simulink model "ControlVehiculoV"  (R2023b)
settings: Solver=FixedStepAuto  StartTime=0.0  StopTime=10  RelTol=1e-3  EnableMultiTasking=on
model workspace (MAT data in the model file):
  d = 0.223
settings Model: ExtModeTrigDuration=2  Creator=Manuel  LastModifiedBy=Manuel
settings OptimizationCC: EnhancedBackFolding=on  PassReuseOutputArgsAs=Individual arguments  ZeroExternalMemoryAtStartup=off  ZeroInternalMemoryAtStartup=off  MaxStackSize=64  OptimizeBlockOrder=speed  DifferentSizesBufferReuse=on  OptimizationCustomize=off  EfficientTunableParamExpr=on
settings DebuggingCC: ParameterTunabilityLossMsg=error
settings HardwareCC: ProdBitPerInt=16  ProdBitPerPointer=16  ProdBitPerSizeT=16  ProdBitPerPtrDiffT=16  ProdLargestAtomicFloat=None  ProdWordSize=8  ProdHWDeviceType=Atmel->AVR
settings SFSimCC: MATLABDynamicMemAlloc=off
settings RTWCC: Description=Embedded Coder  SystemTargetFile=ert.tlc  HardwareBoard=Arduino Mega 2560  TemplateMakefile=ert_default_tmf  Toolchain=Arduino AVR  BuildConfiguration=Faster Runs
settings CodeAppCC: ForceParamTrailComments=on  IgnoreCustomStorageClasses=off  OperatorAnnotations=on  SimulinkDataObjDesc=on  SFDataObjDesc=on  InsertBlockDesc=on
settings ERTTargetCC: SupportContinuousTime=on  SupportVariableSizeSignals=on  ExtModeTransport=3  ExtModeStaticAlloc=on  ExtModeAutomaticAllocSize=off  ExtModeStaticAllocSize=2048  ExtModeMexFile=ext_xcp  ExtModeIntrfLevel=Level2 - Open

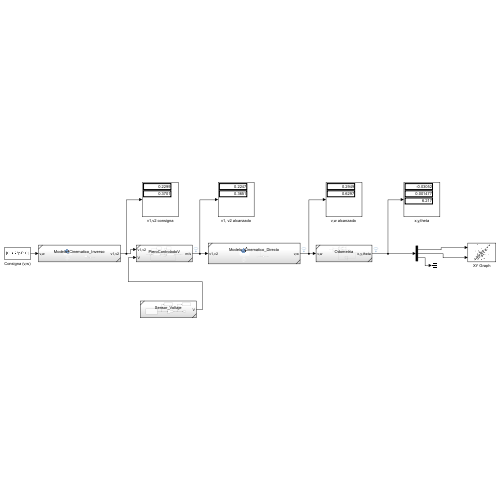
[thumbnail: Simulink's stored preview of the top-level diagram]
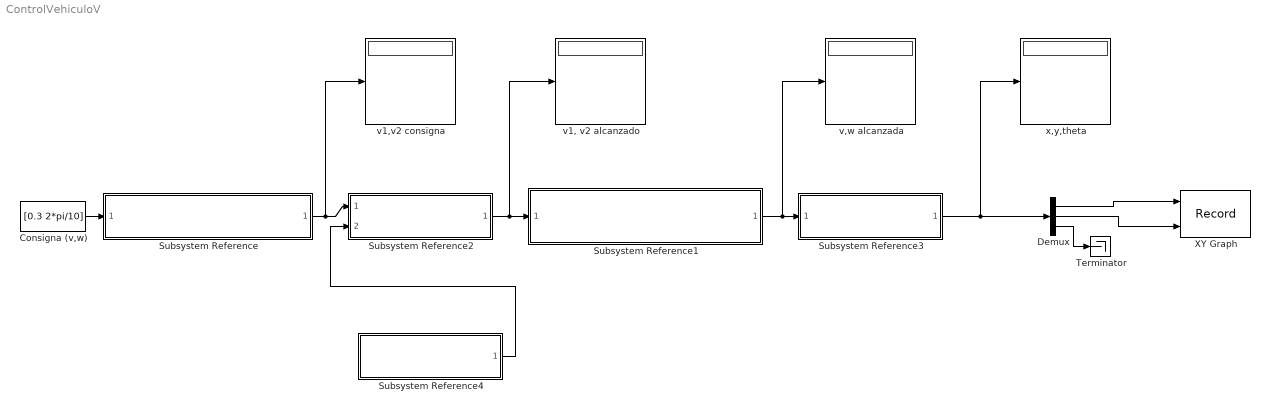
== system ControlVehiculoV ==
  Consigna (v,w) : Constant  Value=[0.3 2*pi/10]
  Demux : Demux  Outputs=3
  Subsystem Reference : Subsystem  ReferencedSubsystem=Modelo_Cinematico_Inverso
  Subsystem Reference1 : Subsystem  ReferencedSubsystem=Modelo_Cinematico_Directo
  Subsystem Reference2 : Subsystem  ReferencedSubsystem=PieroControladoV
  Subsystem Reference3 : Subsystem  ReferencedSubsystem=Odometria
  Subsystem Reference4 : Subsystem  ReferencedSubsystem=Sensor_Voltaje
  Terminator : Terminator
  XY Graph : Record  FileSettingsInternal="{\"entries\":[{\"content\":{\"excelSettings\":{\"content\":{},\"type\":\"Streamout.ExcelSettings\"}},\"type\":\"Streamout.FileSettingStorage\",\"uuid\":\"\"}],\"packageUris\":[\"http:\\/\\/schema.mathworks.com\\/mf0\\/streamout_blocks\\/R2020a\"],\"version\":\"1.0\"}"  Layout=[1 1]  SignalsInternal="{\"entries\":[{\"content\":{\"signals\":[{\"content\":{\"blockPath\":[],\"dimensions\":[1],\"domain\":\"\",\"lineColor\":\"#a2142f\",\"plots\":[1],\"port\":1,\"sid\":[\"16\"],\"signalID\":325284,\"signalName\":\"Demux:1\"},\"type\":\"RecordBlkView.Signal\",\"uuid\":\"\"},{\"content\":{\"blockPath\":[],\"dimensions\":[1],\"domain\":\"\",\"lineColor\":\"#139fff\",\"plots\":[1],\"port\":2,\"sid\":[\"16\"],\"signalID\":325288,\"signalName\":\"Demux:2\"},\"type\":\"RecordBlkView.Signal\",\"uuid\":\"\"}]},\"type\":\"RecordBlkView.InputSignals\",\"uuid\":\"\"}],\"packageUris\":[\"http:\\/\\/schema.mathworks.com\\/mf0\\/streamout_blocks\\/R2020a\"],\"version\":\"1.0\"}"  VisualizationBindings="{\"xyplotplugin\":{\"info\":[{\"series\":[{\"bindingParametersList\":[{\"parameter\":\"X-Axis\",\"signalID\":325284,\"signalName\":\"Demux:1\"},{\"parameter\":\"Y-Axis\",\"signalID\":325288,\"signalName\":\"Demux:2\"}],\"seriesID\":8516}],\"subplotID\":1}]}}"  CompatibilityTag=XY
  "v,w alcanzada " : Display
  "v1, v2 alcanzado" : Display
  v1,v2 consigna : Display
  x,y,theta : Display
  wires:
  Consigna (v,w)/1 -> Subsystem Reference/1
  Subsystem Reference1/1 -> "v,w alcanzada "/1, Subsystem Reference3/1
  Subsystem Reference/1 -> v1,v2 consigna/1, Subsystem Reference2/1
  Subsystem Reference2/1 -> "v1, v2 alcanzado"/1, Subsystem Reference1/1
  Subsystem Reference3/1 -> Demux/1, x,y,theta/1
  Demux/1 -> XY Graph/1
  Demux/2 -> XY Graph/2
  Demux/3 -> Terminator/1
  Subsystem Reference4/1 -> Subsystem Reference2/2
